simulink model "HallSensorTest"  (R2015a)
settings: Solver=ode1  StartTime=0.0  StopTime=Inf  FixedStep=0.001  RelTol=1e-3
PostLoadFcn:
  | , if any(exist('dsrtsu_mdlpostloadfcn', 'file') == [2, 3, 6]), try dsrtsu_mdlpostloadfcn('Execute', bdroot); catch fprintf('Error in PostLoadFcn (dsrtsu_mdlpostloadfcn) for model "%s":\n %s\n', bdroot, lasterr); end, end,
libraries: rti1401lib_dio_type3 x3, rti1401lib_adc_type4 x2, rtilib1401 x1
settings Model: DSRTSU_INTERNAL_RTI_VER=470  DSRTSU_INTERNAL_RTI_TYPE=rti1401  DSRTSU_INTERNAL_RTIFPGA=60  Creator=Powertrain_software  LastModifiedBy=Powertrain_software
settings OptimizationCC: BlockReduction=off  OptimizeBlockIOStorage=off  BufferReuse=off  GlobalBufferReuse=off  ExpressionFolding=off  LocalBlockOutputs=off
settings HardwareCC: ProdLargestAtomicInteger=Integer  ProdLargestAtomicFloat=Float  ProdIntDivRoundTo=Zero  ProdEndianess=BigEndian  ProdHWDeviceType=Generic->Custom  TargetIntDivRoundTo=Zero  TargetEndianess=BigEndian  TargetHWDeviceType=Generic->Custom
settings RTWCC: SystemTargetFile=rti1401.tlc  MakeCommand=make_rti  TemplateMakefile=rti1401.tmf  Description=dSPACE DS1401 Hardware Platform
settings STFCustomTargetCC: GenerateSampleERTMain=off  ParMdlRefBuildCompliant=on  GeneratePreprocessorConditionals=Disable all  ERTCustomFileBanners=off  SupportNonInlinedSFcns=on  SupportVariableSizeSignals=off  MATLABClassNameForMDSCustomization=Simulink.SoftwareTarget.GRTCustomization  GRTInterface=on  SystemTargetFile=rti1401.tlc
settings GRTTargetCC: CompOptLevelCompliant=off  ConcurrentExecutionCompliant=off  CombineOutputUpdateFcns=off  MatFileLogging=off  CPPClassGenCompliant=off  GRTInterface=on  ExtModeMexFile=noextcomm

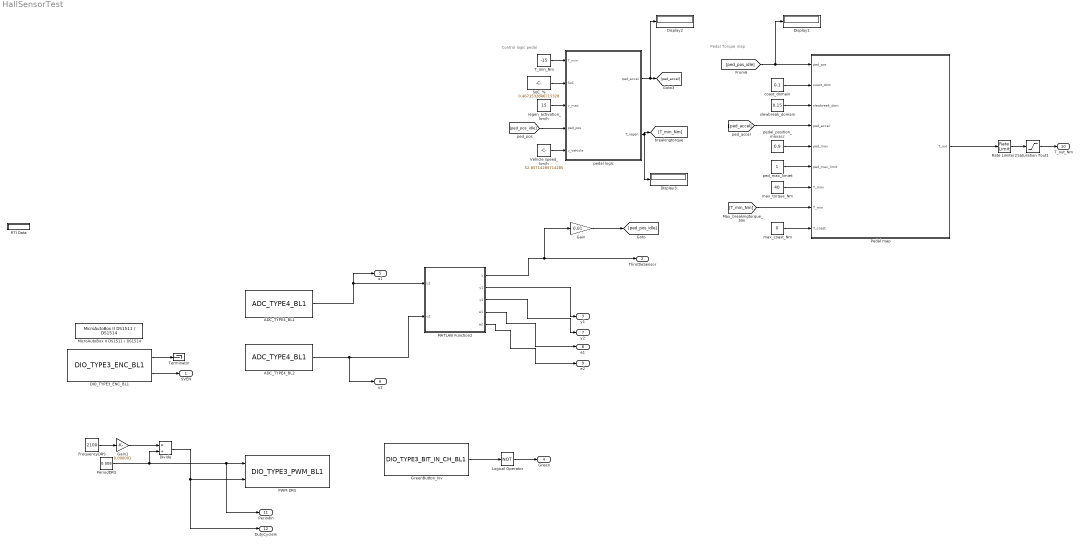
== system HallSensorTest ==
  note: Control logic pedal
  note: Pedal Torque map
  ADC_TYPE4_BL1 : rti1401lib_adc_type4/ADC_TYPE4_BL1  DSProperties=struct('RTI',struct('Version',uint32(2),'BlockType',struct('isSLSource',uint8(1),'isSLSink',uint8(1),'isHWSource',uint8(0),'isHWSink',uint8(1),'isSetup',uint8(0),'isInline',uint8(1),'isNonInline',uint8(0),'isInterrupt',uint8(0),'isChannelwise',uint8(1)),'IOBoardType',{{'DS1401','STD','ADCT4'}},'UnitType','ADC','Identifier','ADC','DialogType','ML','BlockSet','NONE','SlaveProcessor','NONE'))  RTIBlockInterface=struct('InputPortsActive',0,'InputPortsWidth',int32(1),'InputPortsDataType',{{'SS_BOOLEAN'}},'InputPortsName',{{'Continue'}},'OutputPortsActive',[1 0],'OutputPortsWidth',int32([1 1]),'OutputPortsDataType',{{'SS_DOUBLE','SS_UINT8'}},'OutputPortsName',{{'ADC','Status'}},'DialogFcn','rti1401stdadct4adcgui','SampleTime',{{-1}},'InitLevel',3,'IconTransparency','on','BlockDisplay',{{['ADC TP4\nModule: 1\nChannel: 1'],'center'}},'BlockName',struct('Token',{{'ADC_TYPE4_BL1'}}))  RTIBlockParameters=struct('ADCSWStartDisable',{{0,'OFF',[0 1]}},'ModuleNo',{{1,'OFF',[1 16]}},'ChannelNo',{{1,'OFF',[1 16]}},'ConversionMode',{{1,'OFF',[1 2]}},'SampleMode',{{1,'OFF',[1 2]}},'TriggerSource',{{1,'OFF',[1 5]}},'EdgePolarity',{{1,'OFF',[1 2]}},'ConversionTriggerSource',{{2,'OFF',[1 6]}},'ConversionEdgePolarity',{{1,'OFF',[1 2]}},'ConversionPeriod',{{1e-06,'OFF',[]}},'ConversionPeriodCheck',{{0,'OFF',[]}},'BurstTriggerSource',{{1,'OFF',[1 6]}},'BurstEdgePolarity',{{1,'OFF',[1 2]}},'BurstSize',{{10,'OFF',[]}},'BurstSizeCheck',{{0,'OFF',[]}},'DataSetOffset',{{0,'OFF',[]}},'DataSetOffsetCheck',{{0,'OFF',[]}},'DataSetLength',{{1,'OFF',[]}},'DataSetLengthCheck',{{0,'OFF',[]}},'ReadMode',{{1,'OFF',[1 2]}},'SampleTime',{{-1,'OFF',[-1 inf]}},'SampleTimeCheck',{{1,'OFF',[]}},'StatusPortEnable',{{0,'OFF',[0 1]}},'VoltageRange',{{1,'OFF',[1 2]}},'TLCFileName',{{'rti1401adc_t4_adc','OFF',[]}})  RTISFcnParameters=struct('ADCSWStartDisable','int32','ModuleNo','int32','ChannelNo','int16','ConversionMode','int16','SampleMode','int16','TriggerSource','int16','EdgePolarity','int16','ConversionTriggerSource','int16','ConversionEdgePolarity','int16','ConversionPeriod','double','BurstTriggerSource','int16','BurstEdgePolarity','int16','BurstSize','int16','DataSetOffset','int16','DataSetLength','int16','ReadMode','int16','SampleTime','double','StatusPortEnable','int16','VoltageRange','int16','TLCFileName','char')  RTIBlockParaDefault=struct('ADCSWStartDisable',0,'ModuleNo',1,'ChannelNo',1,'ConversionMode',1,'SampleMode',1,'TriggerSource',1,'EdgePolarity',1,'ConversionTriggerSource',2,'ConversionEdgePolarity',1,'ConversionPeriod',1e-06,'ConversionPeriodCheck',0,'BurstTriggerSource',1,'BurstEdgePolarity',1,'BurstSize',10,'BurstSizeCheck',0,'DataSetOffset',0,'DataSetOffsetCheck',0,'DataSetLength',1,'DataSetLengthCheck',0,'ReadMode',1,'SampleTime',-1,'SampleTimeCheck',1,'StatusPortEnable',0,'VoltageRange',1,'TLCFileName','rti1401adc_t4_adc')
  ADC_TYPE4_BL2 : rti1401lib_adc_type4/ADC_TYPE4_BL1  DSProperties=struct('RTI',struct('Version',uint32(2),'BlockType',struct('isSLSource',uint8(1),'isSLSink',uint8(1),'isHWSource',uint8(0),'isHWSink',uint8(1),'isSetup',uint8(0),'isInline',uint8(1),'isNonInline',uint8(0),'isInterrupt',uint8(0),'isChannelwise',uint8(1)),'IOBoardType',{{'DS1401','STD','ADCT4'}},'UnitType','ADC','Identifier','ADC','DialogType','ML','BlockSet','NONE','SlaveProcessor','NONE'))  RTIBlockInterface=struct('InputPortsActive',0,'InputPortsWidth',int32(1),'InputPortsDataType',{{'SS_BOOLEAN'}},'InputPortsName',{{'Continue'}},'OutputPortsActive',[1 0],'OutputPortsWidth',int32([1 1]),'OutputPortsDataType',{{'SS_DOUBLE','SS_UINT8'}},'OutputPortsName',{{'ADC','Status'}},'DialogFcn','rti1401stdadct4adcgui','SampleTime',{{-1}},'InitLevel',3,'IconTransparency','on','BlockDisplay',{{['ADC TP4\nModule: 1\nChannel: 5'],'center'}},'BlockName',struct('Token',{{'ADC_TYPE4_BL1'}}))  RTIBlockParameters=struct('ADCSWStartDisable',{{0,'OFF',[0 1]}},'ModuleNo',{{1,'OFF',[1 16]}},'ChannelNo',{{5,'OFF',[1 16]}},'ConversionMode',{{1,'OFF',[1 2]}},'SampleMode',{{1,'OFF',[1 2]}},'TriggerSource',{{1,'OFF',[1 5]}},'EdgePolarity',{{1,'OFF',[1 2]}},'ConversionTriggerSource',{{2,'OFF',[1 6]}},'ConversionEdgePolarity',{{1,'OFF',[1 2]}},'ConversionPeriod',{{'1e-06','OFF',[]}},'ConversionPeriodCheck',{{0,'OFF',[]}},'BurstTriggerSource',{{1,'OFF',[1 6]}},'BurstEdgePolarity',{{1,'OFF',[1 2]}},'BurstSize',{{'10','OFF',[]}},'BurstSizeCheck',{{0,'OFF',[]}},'DataSetOffset',{{'0','OFF',[]}},'DataSetOffsetCheck',{{0,'OFF',[]}},'DataSetLength',{{'1','OFF',[]}},'DataSetLengthCheck',{{0,'OFF',[]}},'ReadMode',{{1,'OFF',[1 2]}},'SampleTime',{{'-1','OFF',[-1 inf]}},'SampleTimeCheck',{{1,'OFF',[]}},'StatusPortEnable',{{0,'OFF',[0 1]}},'VoltageRange',{{1,'OFF',[1 2]}},'TLCFileName',{{'rti1401adc_t4_adc','OFF',[]}})  RTISFcnParameters=struct('ADCSWStartDisable','int32','ModuleNo','int32','ChannelNo','int16','ConversionMode','int16','SampleMode','int16','TriggerSource','int16','EdgePolarity','int16','ConversionTriggerSource','int16','ConversionEdgePolarity','int16','ConversionPeriod','double','BurstTriggerSource','int16','BurstEdgePolarity','int16','BurstSize','int16','DataSetOffset','int16','DataSetLength','int16','ReadMode','int16','SampleTime','double','StatusPortEnable','int16','VoltageRange','int16','TLCFileName','char')  RTIBlockParaDefault=struct('ADCSWStartDisable',0,'ModuleNo',1,'ChannelNo',1,'ConversionMode',1,'SampleMode',1,'TriggerSource',1,'EdgePolarity',1,'ConversionTriggerSource',2,'ConversionEdgePolarity',1,'ConversionPeriod',1e-06,'ConversionPeriodCheck',0,'BurstTriggerSource',1,'BurstEdgePolarity',1,'BurstSize',10,'BurstSizeCheck',0,'DataSetOffset',0,'DataSetOffsetCheck',0,'DataSetLength',1,'DataSetLengthCheck',0,'ReadMode',1,'SampleTime',-1,'SampleTimeCheck',1,'StatusPortEnable',0,'VoltageRange',1,'TLCFileName','rti1401adc_t4_adc')
  DIO_TYPE3_ENC_BL1 : rti1401lib_dio_type3/DIO_TYPE3_ENC_BL1  DSProperties=struct('RTI',struct('Version',uint32(2),'BlockType',struct('isSLSource',uint8(1),'isSLSink',uint8(0),'isHWSource',uint8(1),'isHWSink',uint8(0),'isSetup',uint8(0),'isInline',uint8(1),'isNonInline',uint8(0),'isInterrupt',uint8(0),'isChannelwise',uint8(1)),'IOBoardType',{{'DS1401','STD','DIOT3'}},'UnitType','ENC','Identifier','ENC','DialogType','ML','BlockSet','NONE','SlaveProcessor','NONE'))  RTIBlockInterface=struct('OutputPortsWidth',int32([1 1]),'OutputPortsActive',[1 1],'OutputPortsName',{{'Position','Speed'}},'BlockDisplay',{{['DIO TP3 ENCODER\nModule: 1\nPort: 1\nChannel: 3'],'center'}},'IconTransparency','on','InitLevel',3,'DialogFcn','rti1401stddiot3encgui','BlockName',struct('Token',{{'DIO_TYPE3_ENC_BL1'}}))  RTIBlockParameters=struct('ModuleNo',{{1,'OFF',[1 16]}},'PortNo',{{1,'OFF',[1 3]}},'ChannelNo',{{3,'OFF',[1 15]}},'MinPosValue',{{'-2097152','ON',[-2097152 2097151.5]}},'MaxPosValue',{{'2097151.75','ON',[-2097151.75 2097151.75]}},'InitPosValue',{{'0','ON',[-2097152 2097151.75]}},'IndexSetMode',{{1,'OFF',[1 3]}},'IndexPosValue',{{'0','ON',[-2097152 2097151.75]}},'IndexGateMode',{{0,'OFF',[0 1]}},'NoiseFilter',{{1,'OFF',[1 8]}},'BuildCheckIndexMode',{{0,'OFF',[0 1]}},'TLCFileName',{{'rti1401dio_t3_enc','OFF',[]}},'EnableInterrupt',{{0,'OFF',[0 1]}},'TriggerEdgeType',{{1,'OFF',[1 3]}})  RTISFcnParameters=struct('ModuleNo','int32','PortNo','int16','ChannelNo','int16','MinPosValue','double','MaxPosValue','double','InitPosValue','double','IndexSetMode','int16','IndexPosValue','double','IndexGateMode','int16','NoiseFilter','int16','BuildCheckIndexMode','int16','TLCFileName','char','EnableInterrupt','int16','TriggerEdgeType','int32')  RTIBlockParaDefault=struct('ModuleNo',1,'PortNo',1,'ChannelNo',1,'MinPosValue',-2097152,'MaxPosValue',2097151.75,'InitPosValue',0,'IndexSetMode',1,'IndexPosValue',0,'IndexGateMode',0,'NoiseFilter',1,'BuildCheckIndexMode',0,'TLCFileName','rti1401dio_t3_enc','EnableInterrupt',0,'TriggerEdgeType',1)
  Display1 : Display
  Display2 : Display
  Display3 : Display
  Divide : Product  Inputs=*/
  FrequencyDRS : Constant  Value=2100
  Gain : Gain  Gain=0.01
  Gain1 : Gain  Gain=0.000001
  GreenButton_Inv : rti1401lib_dio_type3/DIO_TYPE3_BIT_IN_CH_BL1  DSProperties=struct('RTI',struct('Version',uint32(2),'BlockType',struct('isSLSource',uint8(1),'isSLSink',uint8(0),'isHWSource',uint8(1),'isHWSink',uint8(0),'isSetup',uint8(0),'isInline',uint8(1),'isNonInline',uint8(0),'isInterrupt',uint8(0),'isChannelwise',uint8(1)),'IOBoardType',{{'DS1401','STD','DIOT3'}},'UnitType','BIT','Identifier','BITINCH','DialogType','ML','BlockSet','NONE','SlaveProcessor','NONE'))  RTIBlockInterface=struct('OutputPortsWidth',int32(1),'OutputPortsDataType',{{'SS_BOOLEAN'}},'OutputPortsActive',1,'OutputPortsName',{{'Out'}},'BlockDisplay',{{['DIO TP3 BIT IN\n Channelwise\nModule: 1\nPort: 1\nChannel: 1'],'center'}},'IconTransparency','on','InitLevel',3,'DialogFcn','rti1401stddiot3bitinchgui','BlockName',struct('Token',{{'DIO_TYPE3_BIT_IN_CH_BL1'}}))  RTIBlockParameters=struct('ModuleNo',{{1,'OFF',[1 16]}},'PortNo',{{1,'OFF',[1 3]}},'ChannelNo',{{1,'OFF',[1 16]}},'TLCFileName',{{'rti1401dio_t3_bit_in_ch','OFF',[]}},'EnableInterrupt',{{0,'OFF',[0 1]}},'TriggerEdgeType',{{1,'OFF',[1 3]}})  RTISFcnParameters=struct('ModuleNo','int32','PortNo','int16','ChannelNo','int16','TLCFileName','char','EnableInterrupt','int16','TriggerEdgeType','int32')  RTIBlockParaDefault=struct('ModuleNo',1,'PortNo',1,'ChannelNo',1,'TLCFileName','rti1401dio_t3_bit_in_ch','EnableInterrupt',0,'TriggerEdgeType',1)
  Logical Operator : Logic  Operator=NOT  AllPortsSameDT=off  OutDataTypeStr=boolean
  MATLAB Function2 : MATLAB Function  TreatAsAtomicUnit=on
  MicroAutoBox II DS1511 / DS1514 : rtilib1401/MicroAutoBox II DS1511 // DS1514  SystemSampleTime=-1
  PWM DRS : rti1401lib_dio_type3/DIO_TYPE3_PWM_BL1  DSProperties=struct('RTI',struct('Version',uint32(2),'BlockType',struct('isSLSource',uint8(0),'isSLSink',uint8(1),'isHWSource',uint8(0),'isHWSink',uint8(1),'isSetup',uint8(0),'isInline',uint8(1),'isNonInline',uint8(0),'isInterrupt',uint8(0),'isChannelwise',uint8(1)),'IOBoardType',{{'DS1401','STD','DIOT3'}},'UnitType','PWM','Identifier','PWM','DialogType','ML','BlockSet','NONE','SlaveProcessor','NONE'))  RTIBlockInterface=struct('InputPortsWidth',int32([1 1]),'InputPortsActive',[1 1],'InputPortsName',{{'Period',['Duty Cycle']}},'BlockDisplay',{{['DIO TP3 PWM\nModule: 1\nPort: 1\nChannel: 7'],'center'}},'IconTransparency','on','InitLevel',3,'DialogFcn','rti1401stddiot3pwmgui','BlockName',struct('Token',{{'DIO_TYPE3_PWM_BL1'}}))  RTIBlockParameters=struct('ModuleNo',{{1,'OFF',[1 16]}},'PortNo',{{1,'OFF',[1 3]}},'ChannelNo',{{7,'OFF',[1 16]}},'SupplyRailsCh',{{[1 1],'OFF',[0 1 0 1]}},'UpdateMode',{{1,'ON',[1 2]}},'PeriodRange',{{7,'OFF',[1 16]}},'DutyCycleInit',{{'0','OFF',[0 1]}},'PeriodInit',{{'5e-05','OFF',[]}},'TerminationMode',{{0,'OFF',[0 1]}},'OutputTermValidate',{{0,'OFF',[0 1]}},'OutputTermBuildCheck',{{0,'OFF',[]}},'DutyCycleTerm',{{'0','OFF',[0 1]}},'PeriodTerm',{{'5e-05','OFF',[]}},'TLCFileName',{{'rti1401dio_t3_pwm','OFF',[]}},'EnableInterrupt',{{0,'OFF',[0 1]}},'TriggerEdgeType',{{1,'OFF',[1 3]}})  RTISFcnParameters=struct('ModuleNo','int32','PortNo','int16','ChannelNo','int16','SupplyRailsCh','int16','UpdateMode','int16','PeriodRange','int16','DutyCycleInit','double','PeriodInit','double','TerminationMode','int16','OutputTermValidate','int16','DutyCycleTerm','double','PeriodTerm','double','TLCFileName','char','EnableInterrupt','int16','TriggerEdgeType','int32')  RTIBlockParaDefault=struct('ModuleNo',1,'PortNo',1,'ChannelNo',1,'SupplyRailsCh',[1 1],'UpdateMode',1,'PeriodRange',7,'DutyCycleInit',0,'PeriodInit',5e-05,'TerminationMode',0,'OutputTermValidate',0,'OutputTermBuildCheck',0,'DutyCycleTerm',0,'PeriodTerm',5e-05,'TLCFileName','rti1401dio_t3_pwm','EnableInterrupt',0,'TriggerEdgeType',1)
  Pedal map : MATLAB Function  TreatAsAtomicUnit=on
  PeriodDRS : Constant  Value=0.008
  RTI Data : Subsystem  Tag=struct('RTIDataServer',struct('RTIDataServerVs','2','RTIModelDescription','struct(''main'',''HallSensorTest'',''sub'','''',''isMp'',0)'))  LoadFcn="if exist('rtidc'), try,  rtidc('DataHostBlockClbLoad', gcbh); catch, disp(['Warning: ''LoadFcn'' for RTI Data block failed: ' lasterr]); end, end,"  mask(RTI_DATA_HOST){}
      mask help:
      | RTI Data Block.
      | This block is used by RTI to store internal model-dependent data.
      | Please keep this block on the root level of the model. Deleting this block will result in data loss.
      |
      | NEVER DELETE OR COPY THIS BLOCK!
      settings: CopyFcn="if exist('rtidc'), try,  rtidc('DataHostBlockClbCopy', gcbh); catch, disp(['Warning: ''CopyFcn'' for RTI Data block failed: ' lasterr]); end, end,"  DeleteFcn="if exist('rtidc'), try,  rtidc('DataHostBlockClbDelete', gcbh); catch, disp(['Warning: ''DeleteFcn'' for RTI Data block failed: ' lasterr]); end, end,"  ModelCloseFcn="if exist('rtidc'), try,  rtidc('DataHostBlockClbModelClose', gcbh); catch, disp(['Warning: ''ModelCloseFcn'' for RTI Data block failed: ' lasterr]); end, end,"  PreSaveFcn="if exist('rtidc'), try,  rtidc('DataHostBlockClbPreSave', gcbh); catch, disp(['Warning: ''PreSaveFcn'' for RTI Data block failed: ' lasterr]); end, end,"  PostSaveFcn="if exist('rtidc'), try,  rtidc('DataHostBlockClbPostSave', gcbh); catch, disp(['Warning: ''PostSaveFcn'' for RTI Data block failed: ' lasterr]); end, end,"  NameChangeFcn="if exist('rtidc'), try,  rtidc('DataHostBlockClbNameChange', gcbh); catch, disp(['Warning: ''NameChangeFcn'' for RTI Data block failed: ' lasterr]); end, end,"
      mask Help:
      | RTI Data Block.
      | This block is used by RTI to store internal model-dependent data.
      | Please keep this block on the root level of the model. Deleting this block will result in data loss.
      | 
      | NEVER DELETE OR COPY THIS BLOCK!
      mask Display:
      | text(0.5, 0.5, 'RTI Data', 'HorizontalAlignment', 'center');
      | plot([1 0]);
  Rate Limiter2 : RateLimiter  RisingSlewLimit=2000  FallingSlewLimit=-2000  SampleTimeMode=inherited
  Saturation Tout1 : Saturate  UpperLimit=40  LowerLimit=-40
  SoC_% : Constant  Value=0.4671532846715328
  T_min_Nm : Constant  Value=-15
  Terminator : Terminator
  Vehicle speed_km/h : Constant  Value=52.85714285714285
  coast_domain : Constant  Value=0.1
  max_coast_Nm : Constant  Value=0
  max_torque_Nm : Constant  Value=40
  ped_max_limiet : Constant
  pedal logic : Stateflow chart  TreatAsAtomicUnit=on
  pedal_position_maxacc : Constant  Value=0.9
  regen_activation_km/h : Constant  Value=15
  slewbreak_domain : Constant  Value=0.15
  SVEN : Outport
  ThrottleSensor : Outport  Port=2
  y1 : Outport  Port=3
  Green : Outport  Port=4
  u1 : Outport  Port=5
  u2 : Outport  Port=6
  y2 : Outport  Port=7
  e1 : Outport  Port=8
  e2 : Outport  Port=9
  T_out_Nm : Outport  Port=10
  PeriodIn : Outport  Port=11
  DutyCycleIn : Outport  Port=12
  wires:
  DIO_TYPE3_ENC_BL1/2 -> SVEN/1
  DIO_TYPE3_ENC_BL1/1 -> Terminator/1
  GreenButton_Inv/1 -> Logical Operator/1
  Logical Operator/1 -> Green/1
  ADC_TYPE4_BL1/1 -> MATLAB Function2/1(u1), u1/1
  ADC_TYPE4_BL2/1 -> MATLAB Function2/2(u2), u2/1
  MATLAB Function2/2(y1) -> y1/1
  MATLAB Function2/3(y2) -> y2/1
  MATLAB Function2/4(e1) -> e1/1
  MATLAB Function2/5(e2) -> e2/1
  Saturation Tout1/1 -> T_out_Nm/1
  Pedal map/1(T_out) -> Rate Limiter2/1
  [ped_accel] -> Pedal map/4(ped_accel)
  Rate Limiter2/1 -> Saturation Tout1/1
  coast_domain/1 -> Pedal map/2(coast_dom)
  Vehicle speed_km/h/1 -> pedal logic/5(v_vehicle)
  [ped_pos_idle] -> pedal logic/4(ped_pos)
  pedal_position_maxacc/1 -> Pedal map/5(ped_max)
  T_min_Nm/1 -> pedal logic/1(T_min)
  ped_max_limiet/1 -> Pedal map/6(ped_max_limit)
  [ped_pos_idle] -> Pedal map/1(ped_pos), Display1/1
  slewbreak_domain/1 -> Pedal map/3(slewbreak_dom)
  [T_min_Nm] -> Pedal map/8(T_min)
  SoC_%/1 -> pedal logic/2(SoC)
  pedal logic/2(T_regen) -> Display3/1, [T_min_Nm]
  max_torque_Nm/1 -> Pedal map/7(T_max)
  pedal logic/1(ped_accel) -> Display2/1, [ped_accel]
  regen_activation_km/h/1 -> pedal logic/3(v_max)
  max_coast_Nm/1 -> Pedal map/9(T_coast)
  MATLAB Function2/1(y) -> Gain/1, ThrottleSensor/1
  Gain/1 -> [ped_pos_idle]
  PeriodDRS/1 -> Divide/2, PeriodIn/1, PWM DRS/1
  FrequencyDRS/1 -> Gain1/1
  Divide/1 -> DutyCycleIn/1, PWM DRS/2
  Gain1/1 -> Divide/1

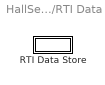
== system HallSensorTest/RTI Data ==
  RTI Data Store : Subsystem  Tag="struct('private',struct('version',struct('dsVer',uint32(2),'dsVerCreation',uint32(2),'RTI',struct('ver','7.5','type','RTI1401')),'access',struct('type','Model','isPerm',1,'created',['11-May-2016 13:41:37'],'modified',['15-May-2016 17:38:29'],'location','')),'public',struct('main',struct('data',[]),'sub',struct('name',{{'HallSensorTest'}},'data',{{struct('TH',struct('thTaskInfo',struct('taskType',{'TIMER','HWINT','TMRINT','SWINT','GLINT'},'tasksNumOf',{1,0,0,0,0},'srcIds',{{'TIMERA'},{},{},{},{}},'taskNames',{{['Timer Task 1']},{},{},{},{}})),'th_tc',struct('dataType','TASK','taskGroupId','','taskGroupList',{{}},'taskSchedulingPolicy','FCFS','taskType','TIMER','blkh',-1,'srcId','TIMERA','srcSgnName',['Timer A interrupt'],'srcCpuName','','taskName',['Timer Task 1  [0.001] s'],'taskNameDisplayExt','','smplTime',0.001,'smplTimeOffs',0,'hasFixedPriority',0,'priority',1,'hasFixedOvc',0,'ovcType',1,'ovcMax',1),'tc_th',struct('dataType','TASK','taskGroupId','','taskGroupList',{{}},'taskSchedulingPolicy','FCFS','taskType','TIMER','blkh',-1,'srcId','TIMERA','srcSgnName',['Timer A interrupt'],'srcCpuName','','taskName',['Timer Task 1  [0.001] s'],'taskNameDisplayExt','','smplTime',0.001,'smplTimeOffs',0,'hasFixedPriority',0,'priority',1,'hasFixedOvc',0,'ovcType',1,'ovcMax',1))}})))"  mask(RTI_DATA_STORE){}
      mask help:
      | RTI Data Store Block. This block is used by RTI to store internal model dependent data. Deleting this block will result in data loss.
      |
      | NEVER DELETE, COPY, OR MODIFY THIS BLOCK!
      mask Help:
      | RTI Data Store Block. This block is used by RTI to store internal model dependent data. Deleting this block will result in data loss.
      | 
      | NEVER DELETE, COPY, OR MODIFY THIS BLOCK!
      mask Display: text(0.5, 0.5, ' ', 'HorizontalAlignment', 'center');

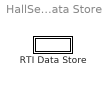
== system HallSensorTest/RTI Data/RTI Data Store ==
  RTI Data Store : Subsystem  mask(RTI_DATA_STORE){}
      mask help:
      | RTI Data Store Block. This block is used by RTI to store internal model dependent data. Deleting this block will result in data loss.
      |
      | NEVER DELETE, COPY, OR MODIFY THIS BLOCK!
      mask Help:
      | RTI Data Store Block. This block is used by RTI to store internal model dependent data. Deleting this block will result in data loss.
      | 
      | NEVER DELETE, COPY, OR MODIFY THIS BLOCK!
      mask Display: text(0.5, 0.5, ' ', 'HorizontalAlignment', 'center');

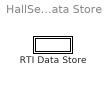
== system HallSensorTest/RTI Data/RTI Data Store/RTI Data Store ==
  RTI Data Store : Subsystem  mask(RTI_DATA_STORE){}
      mask help:
      | RTI Data Store Block. This block is used by RTI to store internal model dependent data. Deleting this block will result in data loss.
      |
      | NEVER DELETE, COPY, OR MODIFY THIS BLOCK!
      mask Help:
      | RTI Data Store Block. This block is used by RTI to store internal model dependent data. Deleting this block will result in data loss.
      | 
      | NEVER DELETE, COPY, OR MODIFY THIS BLOCK!
      mask Display: text(0.5, 0.5, ' ', 'HorizontalAlignment', 'center');

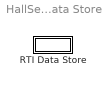
== system HallSensorTest/RTI Data/RTI Data Store/RTI Data Store/RTI Data Store ==
  RTI Data Store : Subsystem  mask(RTI_DATA_STORE){}
      mask help:
      | RTI Data Store Block. This block is used by RTI to store internal model dependent data. Deleting this block will result in data loss.
      |
      | NEVER DELETE, COPY, OR MODIFY THIS BLOCK!
      mask Help:
      | RTI Data Store Block. This block is used by RTI to store internal model dependent data. Deleting this block will result in data loss.
      | 
      | NEVER DELETE, COPY, OR MODIFY THIS BLOCK!
      mask Display: text(0.5, 0.5, ' ', 'HorizontalAlignment', 'center');

== system HallSensorTest/RTI Data/RTI Data Store/RTI Data Store/RTI Data Store/RTI Data Store ==

== matlab function HallSensorTest/Pedal map ==
  data: ped_pos input; coast_dom input; T_out output; slewbreak_dom input; ped_accel input; ped_max input; ped_max_limit input; T_max input; T_min input; T_coast input
function T_out = Pedalmap_eq(ped_pos,coast_dom,slewbreak_dom,ped_accel,ped_max,ped_max_limit,T_max,T_min,T_coast)
%%Accelerator pedal mapping:

ped_regen=ped_accel-coast_dom; %pedal postion - start regen - variable in function of velocity
ped_zero=ped_regen-slewbreak_dom; %pedal postion - start max regen - variable in function of velocity

slewrate_acc=(T_max-T_coast)/(ped_max-ped_accel); %slewrate acceleration region
slewrate_regen=(T_min-T_coast)/(ped_zero-ped_regen);%slewrate regen region

% acceleration pedal map eq.
T_out=T_min*(heavi(ped_pos,0)-heavi(ped_pos,ped_zero)) + (slewrate_regen*(ped_pos-ped_regen)+T_coast)*(heavi(ped_pos,ped_zero)-heavi(ped_pos,ped_regen))+T_coast*(heavi(ped_pos,ped_regen)-heavi(ped_pos,ped_accel))+(slewrate_acc*(ped_pos-ped_accel)+T_coast)*(heavi(ped_pos,ped_accel)-heavi(ped_pos,ped_max))+T_max*(heavi(ped_pos,ped_max-heavi(ped_pos,ped_max_limit)));

== stateflow chart HallSensorTest/pedal logic ==
  state Driving
    state Disable_regen %SoC is to high.
      entry:
      ped_accel=0.45;
      T_regen=0;
    state Activate_regen
      entry:
      ped_accel=0.45;
      T0= -5; %Regentorque at v_max [Nm]
      during:
      % velocity dependant braking torque
      if v_vehicle<15
      T_regen=T_min/15
      elseif v_vehicle<50
      T_regen=T_min
      else
      T_regen=(T_min-T0)/(50-100)*(v_vehicle-100)+T0
      end
    (default) -> Disable_regen %SoC is to high.
    Disable_regen %SoC is to high. -> Activate_regen : [SoC<0.95]
    Activate_regen -> Disable_regen %SoC is to high. : [SoC>0.95]
  state Standstill
    entry:
    T_regen=0;
    ped_accel=0.1; %
    during:
    %velocity dependent coasting until v_max
    if ped_pos>0.1
    ped_accel=min(ped_pos* (v_vehicle/v_max),0.45); %Offset of 0.1
    end
    exit:
    ped_accel=0.45;
  (default) -> Standstill
  Driving -> Standstill : [v_vehicle<=3]
  Standstill -> Driving : [v_vehicle >v_max&&ped_pos>0.45]
  data: T_min input; SoC input; v_max input; ped_pos input; v_vehicle input; ped_accel output; T_regen output; T0 local

== matlab function HallSensorTest/MATLAB Function2 ==
  data: y output; u1 input; u2 input; y1 output; y2 output; e1 output; e2 output
function [y,y1,y2,e1,e2] = ThrottleSensorCalculation(u1, u2)

% Variables
lowerlim1 = 0.33;
upperlim1 = 0.73;
lowerlim2 = 0.30;
upperlim2 = 0.70;

% ThrottleSensor1
t1 = (1-u1);
if t1 < lowerlim1
    y1 = 0;
elseif t1 > upperlim1
    y1 = 1;   
else
    y1 = (1/(upperlim1-lowerlim1))*(t1-lowerlim1);
end

% ThrottleSensor2
t2 = (1-u2);
if t2 < lowerlim2
    y2 = 0;
elseif t2 > upperlim2
    y2 = 1;   
else
    y2 = (1/(upperlim2-lowerlim2))*(t2-lowerlim2);
end

% ErrorCheck
if u1 > 0.10 && u1 < 0.90 && u2 > 0.10 && u2 < 0.90   
    if abs(y1-y2) > 0.10
        e1 = 1;
        e2 = 1;
        y = 0;
    else
        e1 = 0;
        e2 = 0;
        y = (y1+y2)/2;
    end
else
    if (u1 < 0.10 || u1 > 0.90) && (u2 < 0.10 || u2 > 0.90)
        e1 = 1;
        e2 = 1;
        y = 0;
    elseif u1 < 0.10 || u1 > 0.90
        e1 = 1;
        e2 = 0;
        y = y2;
    else
        e1 = 0;
        e2 = 1;
        y = y1;
    end  
    
%     e1 = 1;
%     e2 = 1;
%     y = 0;
end
